simulink model "payload"  (R2024b)
settings: Solver=VariableStepAuto  StartTime=0.0  StopTime=10  FixedStep=0.01  RelTol=1e-3
settings Model: Creator=yangyu  LastModifiedBy=yangyu

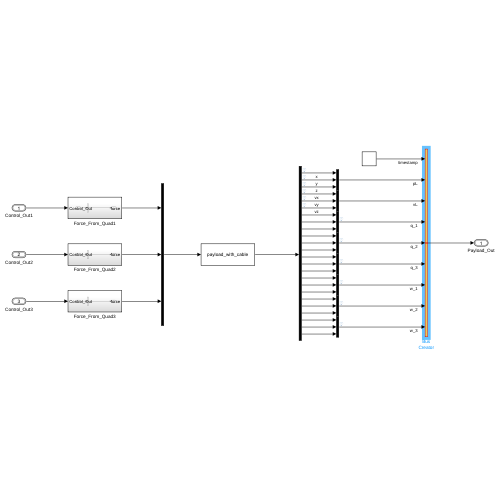
[thumbnail: Simulink's stored preview of the top-level diagram]
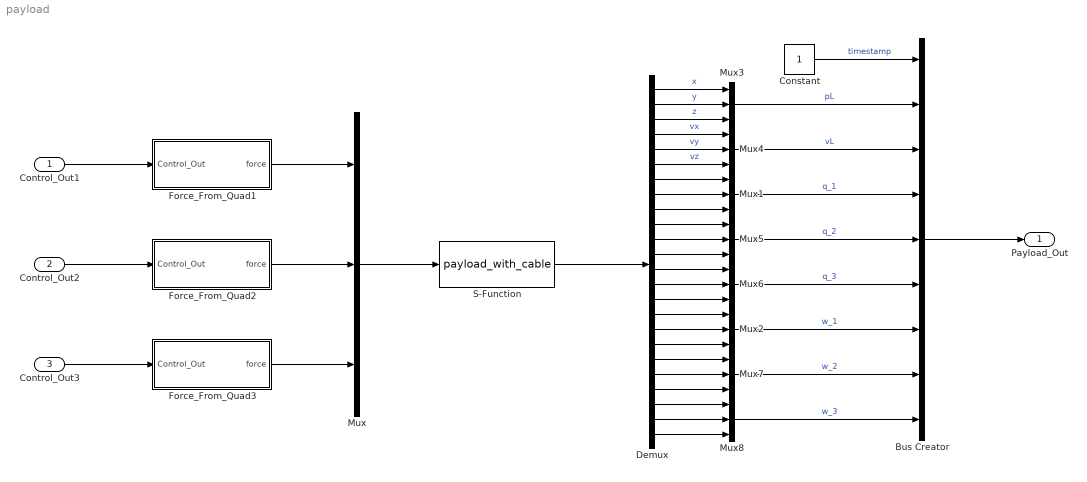
== system payload ==
  Control_Out1 : Inport  OutDataTypeStr=Bus: Control_Out_Bus
  Control_Out2 : Inport  Port=2  OutDataTypeStr=Bus: Control_Out_Bus
  Control_Out3 : Inport  Port=3  OutDataTypeStr=Bus: Control_Out_Bus
  Bus Creator : BusCreator  Inputs=9  OutDataTypeStr=Bus: Payload_Out_Bus
  Constant : Constant  OutDataTypeStr=Inherit: Inherit via back propagation
  Demux : Demux  Outputs=24
  Force_From_Quad1 : Subsystem
  Force_From_Quad2 : Subsystem
  Force_From_Quad3 : Subsystem
  Mux{,1..8} (9 alike) : Mux  Inputs=3
  S-Function : S-Function  FunctionName=payload_with_cable  SFunctionDeploymentMode=off  EnableBusSupport=off
  Payload_Out : Outport  OutDataTypeStr=Bus: Payload_Out_Bus
  wires:
  S-Function/1 -> Demux/1
  Demux/1 -> Mux3/1  "x"
  Demux/2 -> Mux3/2  "y"
  Demux/3 -> Mux3/3  "z"
  Force_From_Quad1/1(force) -> Mux/1
  Demux/4 -> Mux4/1  "vx"
  Demux/5 -> Mux4/2  "vy"
  Demux/6 -> Mux4/3  "vz"
  Demux/7 -> Mux1/1
  Demux/9 -> Mux1/3
  Demux/8 -> Mux1/2
  Demux/11 -> Mux5/2
  Demux/10 -> Mux5/1
  Demux/12 -> Mux5/3
  Demux/13 -> Mux6/1
  Demux/14 -> Mux6/2
  Demux/15 -> Mux6/3
  Demux/24 -> Mux8/3
  Demux/23 -> Mux8/2
  Demux/22 -> Mux8/1
  Demux/21 -> Mux7/3
  Demux/20 -> Mux7/2
  Demux/19 -> Mux7/1
  Mux1/1 -> Bus Creator/4  "q_1"
  Demux/17 -> Mux2/2
  Demux/16 -> Mux2/1
  Demux/18 -> Mux2/3
  Mux2/1 -> Bus Creator/7  "w_1"
  Force_From_Quad2/1(force) -> Mux/2
  Force_From_Quad3/1(force) -> Mux/3
  Mux3/1 -> Bus Creator/2  "pL"
  Mux4/1 -> Bus Creator/3  "vL"
  Mux5/1 -> Bus Creator/5  "q_2"
  Mux6/1 -> Bus Creator/6  "q_3"
  Mux7/1 -> Bus Creator/8  "w_2"
  Mux8/1 -> Bus Creator/9  "w_3"
  Control_Out1/1 -> Force_From_Quad1/1(Control_Out)
  Control_Out2/1 -> Force_From_Quad2/1(Control_Out)
  Control_Out3/1 -> Force_From_Quad3/1(Control_Out)
  Constant/1 -> Bus Creator/1  "timestamp"
  Bus Creator/1 -> Payload_Out/1
  Mux/1 -> S-Function/1

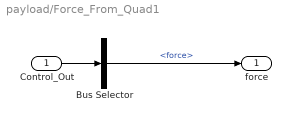
== system payload/Force_From_Quad1 ==
  Control_Out : Inport
  Bus Selector : BusSelector  OutputSignals=force
  force : Outport
  wires:
  Control_Out/1 -> Bus Selector/1
  Bus Selector/1 -> force/1  "<force>"

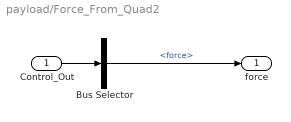
== system payload/Force_From_Quad2 ==
  Control_Out : Inport
  Bus Selector : BusSelector  OutputSignals=force
  force : Outport
  wires:
  Control_Out/1 -> Bus Selector/1
  Bus Selector/1 -> force/1  "<force>"

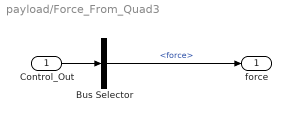
== system payload/Force_From_Quad3 ==
  Control_Out : Inport
  Bus Selector : BusSelector  OutputSignals=force
  force : Outport
  wires:
  Control_Out/1 -> Bus Selector/1
  Bus Selector/1 -> force/1  "<force>"
